simulink model "Simulacion"  (R2020a)
settings: Solver=VariableStepAuto  StartTime=0.0  StopTime=15  RelTol=1e-3
libraries: simulink x2
settings Model: Creator=HP  LastModifiedBy=HP

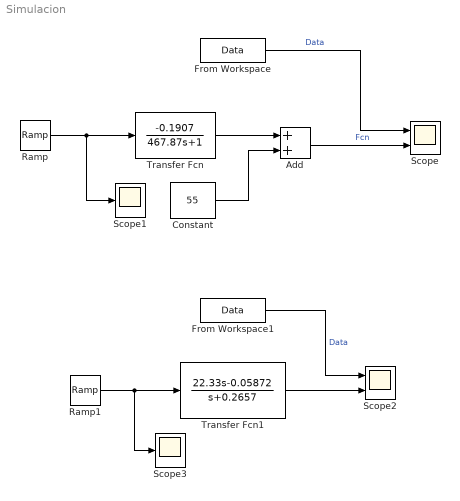
== system Simulacion ==
  Add : Sum
  Constant : Constant  Value=55
  From Workspace : FromWorkspace  VariableName=Data
  From Workspace1 : FromWorkspace  VariableName=Data
  Ramp : simulink/Sources/Ramp  slope=1  start=0  InitialOutput=0
  Ramp1 : simulink/Sources/Ramp  slope=1  start=0  InitialOutput=0  VectorParams1D=off
  Scope : Scope  NumInputPorts=2
  Scope1 : Scope
  Scope2 : Scope  NumInputPorts=2
  Scope3 : Scope
  Transfer Fcn : TransferFcn  Numerator=[-0.1907]  Denominator=[467.87 1]
  Transfer Fcn1 : TransferFcn  Numerator=[22.33 -0.05872]  Denominator=[1 0.2657]
  wires:
  Transfer Fcn/1 -> Add/1
  Constant/1 -> Add/2
  Add/1 -> Scope/2  "Fcn"
  From Workspace/1 -> Scope/1  "Data"
  Transfer Fcn1/1 -> Scope2/2
  From Workspace1/1 -> Scope2/1  "Data"
  Ramp1/1 -> Scope3/1, Transfer Fcn1/1
  Ramp/1 -> Scope1/1, Transfer Fcn/1
